simulink model "pplaceg_c"  (Simulink 5.0)
settings: Solver=ode23s  StartTime=0.0  StopTime=10  RelTol=1e-8  AbsTol=1.0e-8
values from neighbouring files (symbols this model uses):
  a = [0 1 0; a21 0 a23; 0 0 a33]    [ball_basic.m]
  b = [0; 0; b3]    [ball_basic.m]
  c = [1 0 0]    [ball_basic.m]
  d = 0    [ball_basic.m]
  R = 1    [ball_basic.m]    (also in unstb_stb.m)
  Ts = 0.01; [B,A,k] = myc2d(G,Ts)    [ball_basic.m]    (also in unstb_stb.m = 1)
undefined symbols (not defined in the file or in its folder): S, TN
settings Model: Creator=kannanm  LastModifiedBy=kannanm  ExtModeAutoUpdateStatusClock=off

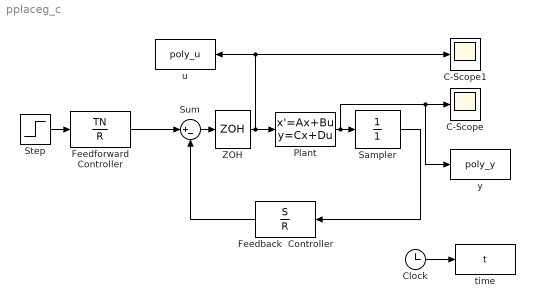
== system pplaceg_c ==
  C-Scope : Scope
      settings: YMin=0  YMax=1.2
  C-Scope1 : Scope
      settings: YMin=0  YMax=1.2
  Clock : Clock
      settings: Decimation=10
  Feedback  Controller : DiscreteFilter  Orientation=left  Numerator=S  Denominator=R  SampleTime=Ts
  Feedforward Controller : DiscreteFilter  Numerator=TN  Denominator=R  SampleTime=Ts
  Plant : StateSpace  A=a  B=b  C=c  D=d  X0=[0 0]
  Sampler : DiscreteFilter  Numerator=1  Denominator=1  SampleTime=Ts
  Step : Step  Time=0  SampleTime=Ts
  Sum : Sum  Inputs=|+-  SaturateOnIntegerOverflow=on
  ZOH : ZeroOrderHold  SampleTime=Ts
  time : ToWorkspace  VariableName=t  SampleTime=Ts  SaveFormat=Array
  u : ToWorkspace  VariableName=poly_u  SampleTime=Ts  SaveFormat=Array
  y : ToWorkspace  VariableName=poly_y  SampleTime=Ts  SaveFormat=Array
  wires:
  Step/1 -> Feedforward Controller/1
  Feedforward Controller/1 -> Sum/1
  Sum/1 -> ZOH/1
  Feedback  Controller/1 -> Sum/2
  Sampler/1 -> Feedback  Controller/1
  Plant/1 -> Sampler/1, C-Scope/1, y/1
  ZOH/1 -> Plant/1, C-Scope1/1, u/1
  Clock/1 -> time/1
